simulink model "Motor_Control_STR"  (R2022a)
settings: Solver=FixedStepDiscrete  StartTime=0.0  StopTime=200  FixedStep=0.005  RelTol=1e-3
libraries: slpidlib x1
settings Model: Creator=PC  LastModifiedBy=dat
settings SolverCC: AlgebraicLoopSolver=TrustRegion
settings DataIOCC: ReturnWorkspaceOutputs=off
settings OptimizationCC: DefaultParameterBehavior=Inlined  PassReuseOutputArgsAs=Individual arguments  EfficientTunableParamExpr=on
settings DebuggingCC: ParameterTunabilityLossMsg=error  UnconnectedInputMsg=warning  UnconnectedOutputMsg=warning  UnconnectedLineMsg=warning  ArithmeticOperatorsInVariantConditions=warning
settings SFSimCC: SimUseLocalCustomCode=off  MATLABDynamicMemAlloc=off  CustomCodeUndefinedFunction=UseInterfaceOnly
settings RTWCC: SystemTargetFile=ert.tlc  GenCodeOnly=on  TemplateMakefile=ert_default_tmf  GenerateReport=on  RTWUseLocalCustomCode=off  IncludeHyperlinkInReport=on  LaunchReport=on  GenerateTraceInfo=on  GenerateTraceReport=on  GenerateTraceReportSl=on  GenerateTraceReportSf=on  GenerateTraceReportEml=on
settings CodeAppCC: ForceParamTrailComments=on  IgnoreCustomStorageClasses=off  OperatorAnnotations=on  SimulinkDataObjDesc=on  SFDataObjDesc=on  InsertBlockDesc=on
settings ERTTargetCC: TargetLangStandard=C99 (ISO)  GenerateSampleERTMain=on  InlinedParameterPlacement=NonHierarchical  ERTCustomFileTemplate=example_file_process.tlc

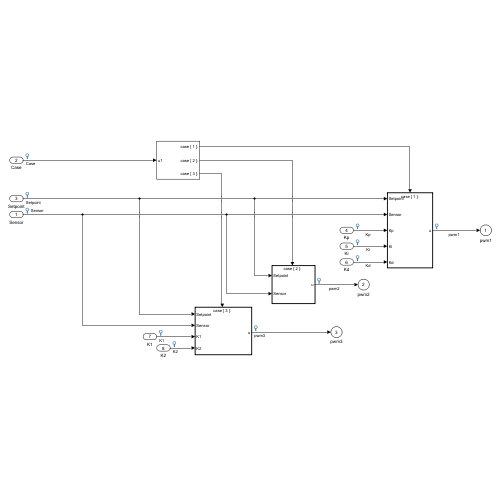
[thumbnail: Simulink's stored preview of the top-level diagram]
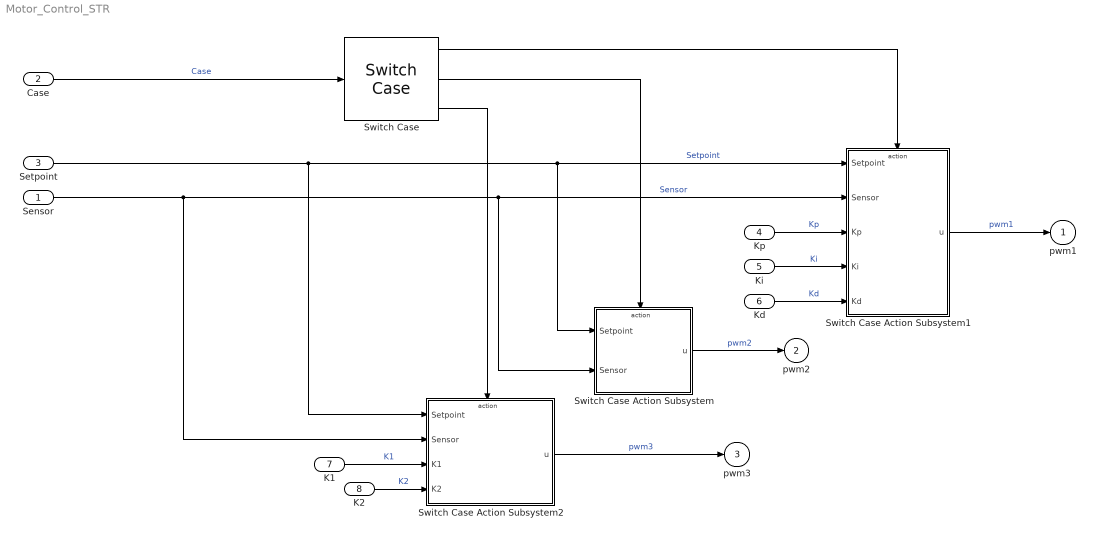
== system Motor_Control_STR ==
  Sensor : Inport
  Case : Inport  Port=2
  Setpoint : Inport  Port=3
  Kp : Inport  Port=4
  Ki : Inport  Port=5
  Kd : Inport  Port=6
  K1 : Inport  Port=7
  K2 : Inport  Port=8
  Switch Case : SwitchCase  CaseConditions={1,2,3}  ShowDefaultCase=off
  Switch Case Action Subsystem : Subsystem  TreatAsAtomicUnit=on
  Switch Case Action Subsystem1 : Subsystem  TreatAsAtomicUnit=on
  Switch Case Action Subsystem2 : Subsystem  TreatAsAtomicUnit=on
  pwm1 : Outport  VectorParamsAs1DForOutWhenUnconnected=off
  pwm2 : Outport  Port=2  VectorParamsAs1DForOutWhenUnconnected=off
  pwm3 : Outport  Port=3  VectorParamsAs1DForOutWhenUnconnected=off
  wires:
  Case/1 -> Switch Case/1  "Case"
  Sensor/1 -> Switch Case Action Subsystem2/2(Sensor), Switch Case Action Subsystem/2(Sensor), Switch Case Action Subsystem1/2(Sensor)  "Sensor"
  Switch Case Action Subsystem1/1(u) -> pwm1/1  "pwm1"
  Switch Case/2 -> Switch Case Action Subsystem/Action
  Switch Case/1 -> Switch Case Action Subsystem1/Action
  Kp/1 -> Switch Case Action Subsystem1/3(Kp)  "Kp"
  Ki/1 -> Switch Case Action Subsystem1/4(Ki)  "Ki"
  Kd/1 -> Switch Case Action Subsystem1/5(Kd)  "Kd"
  Setpoint/1 -> Switch Case Action Subsystem2/1(Setpoint), Switch Case Action Subsystem/1(Setpoint), Switch Case Action Subsystem1/1(Setpoint)  "Setpoint"
  Switch Case Action Subsystem/1(u) -> pwm2/1  "pwm2"
  Switch Case Action Subsystem2/1(u) -> pwm3/1  "pwm3"
  Switch Case/3 -> Switch Case Action Subsystem2/Action
  K2/1 -> Switch Case Action Subsystem2/4(K2)  "K2"
  K1/1 -> Switch Case Action Subsystem2/3(K1)  "K1"

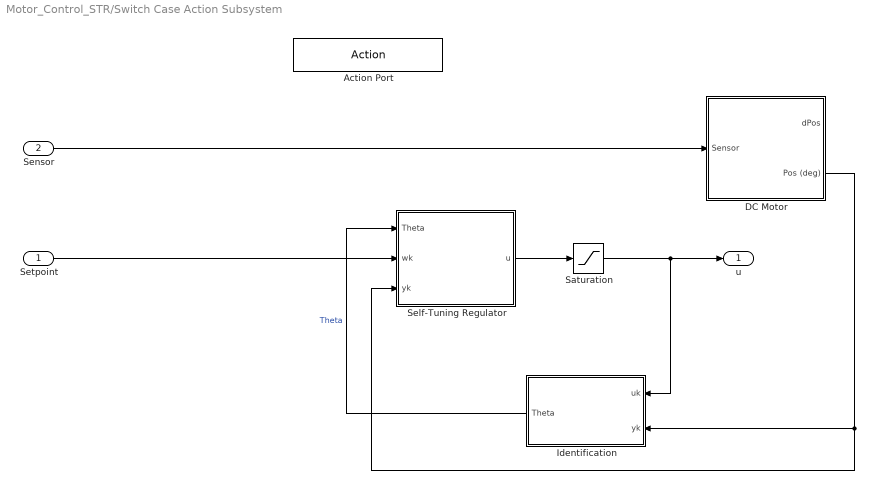
== system Motor_Control_STR/Switch Case Action Subsystem ==
  Setpoint : Inport
  Sensor : Inport  Port=2
  Action Port : ActionPort  ActionPortLabel=case [ 2 ]:
  DC Motor : Subsystem
  Identification : Subsystem
  Saturation : Saturate  UpperLimit=10  LowerLimit=-10
  Self-Tuning Regulator : Subsystem
  u : Outport  VectorParamsAs1DForOutWhenUnconnected=off
  wires:
  Setpoint/1 -> Self-Tuning Regulator/2(wk)
  DC Motor/2(Pos (deg)) -> Self-Tuning Regulator/3(yk), Identification/2(yk)
  Sensor/1 -> DC Motor/1(Sensor)
  Identification/1(Theta) -> Self-Tuning Regulator/1(Theta)  "Theta"
  Self-Tuning Regulator/1(u) -> Saturation/1
  Saturation/1 -> u/1, Identification/1(uk)

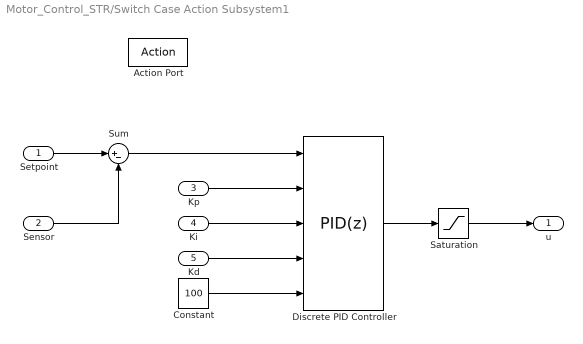
== system Motor_Control_STR/Switch Case Action Subsystem1 ==
  Setpoint : Inport
  Sensor : Inport  Port=2
  Kp : Inport  Port=3
  Ki : Inport  Port=4
  Kd : Inport  Port=5
  Action Port : ActionPort  ActionPortLabel=case [ 1 ]:
  Constant : Constant  Value=100
  Discrete PID Controller : slpidlib/PID Controller  Controller=PID  Form=Parallel  TimeDomain=Discrete-time  UseExternalTs=off  SampleTime=-1  IntegratorMethod=Forward Euler  FilterMethod=Forward Euler  ControllerParametersSource=external  P=1  I=1  UseKiTs=off  D=0  N=100  UseFilter=on  TunerSelectOption=Transfer Function Based (PID Tuner App)  InitialConditionSource=internal  InitialConditionForIntegrator=0  InitialConditionForFilter=0  DifferentiatorICPrevScaledInput=0  ExternalReset=none  TrackingMode=off  Kt=1  LimitOutput=off  SatLimitsSource=internal  UpperSaturationLimit=inf  LowerSaturationLimit=-inf  LinearizeAsGain=off  AntiWindupMode=none  Kb=1  POutMin=[]  POutMax=[]  IOutMin=[]  IOutMax=[]  DOutMin=[]  DOutMax=[]  NOutMin=[]  NOutMax=[]  SumOutMin=[]  SumOutMax=[]  SaturationOutMin=[]  SaturationOutMax=[]  PParamMin=[]  PParamMax=[]  IParamMin=[]  IParamMax=[]  DParamMin=[]  DParamMax=[]  NParamMin=[]  NParamMax=[]  KbParamMin=[]  KbParamMax=[]  KtParamMin=[]  KtParamMax=[]  KbOutMin=[]  KbOutMax=[]  KtOutMin=[]  KtOutMax=[]  IntegratorOutMin=[]  IntegratorOutMax=[]  FilterOutMin=[]  FilterOutMax=[]  SumI1OutMin=[]  SumI1OutMax=[]  SumI2OutMin=[]  SumI2OutMax=[]  SumI3OutMin=[]  SumI3OutMax=[]  SumI4OutMin=[]  SumI4OutMax=[]  SumDOutMin=[]  SumDOutMax=[]  DifferentiatorOutMin=[]  DifferentiatorOutMax=[]  FilterDiffOutCoefMin=[]  FilterDiffOutCoefMax=[]  ReciprocalOutMin=[]  ReciprocalOutMax=[]  SumDenOutMin=[]  SumDenOutMax=[]  SumNumOutMin=[]  SumNumOutMax=[]  DivideOutMin=[]  DivideOutMax=[]  UdiffTsProdOutMin=[]  UdiffTsProdOutMax=[]  NTsProdOutMin=[]  NTsProdOutMax=[]  UintegralTsProdOutMin=[]  UintegralTsProdOutMax=[]  UngainTsProdOutMin=[]  UngainTsProdOutMax=[]  IntegratorContinuousStateAttributes=''  IntegratorStateMustResolveToSignalObject=off  IntegratorRTWStateStorageClass=Auto  FilterContinuousStateAttributes=''  FilterStateMustResolveToSignalObject=off  FilterRTWStateStorageClass=Auto  ParallelPVariant=ExternalParameters  IdealPVariant=Disabled  IVariant=ExternalParameters  DVariant=ExternalParameters  IntegratorVariant=Discrete  SatVariant=Disabled  AWVariant=Passthrough  PCopyVariant=Disabled  TRVariant=Disabled  FdbkBlocksVariant=Forward  IdealPFdbkVariant=Disabled  SatFdbkVariant=Disabled  DerivativeFilterVariant=ForwardEulerFilter  NVariant=ExternalParameters  NCopyVariant=Disabled  FilterICVariant=InternalICsFilter  IntegratorICVariant=InternalICs  ExternalResetVariant=Disabled  TRSumVariant=Passthrough  SumFdbkVariant=Disabled  SumVariant=Sum_PID  TsampFilterVariant=InternalTs  TsampNgainVariant=Passthrough  TsampIntegralVariant=Disabled_SignalSpec  ExternalSaturationOutDataTypeStr=Inherit: Same as second input
  Saturation : Saturate  UpperLimit=10  LowerLimit=-10
  Sum : Sum  Inputs=|+-
  u : Outport  VectorParamsAs1DForOutWhenUnconnected=off
  wires:
  Setpoint/1 -> Sum/1
  Sensor/1 -> Sum/2
  Sum/1 -> Discrete PID Controller/1
  Kp/1 -> Discrete PID Controller/2
  Ki/1 -> Discrete PID Controller/3
  Kd/1 -> Discrete PID Controller/4
  Constant/1 -> Discrete PID Controller/5
  Discrete PID Controller/1 -> Saturation/1
  Saturation/1 -> u/1

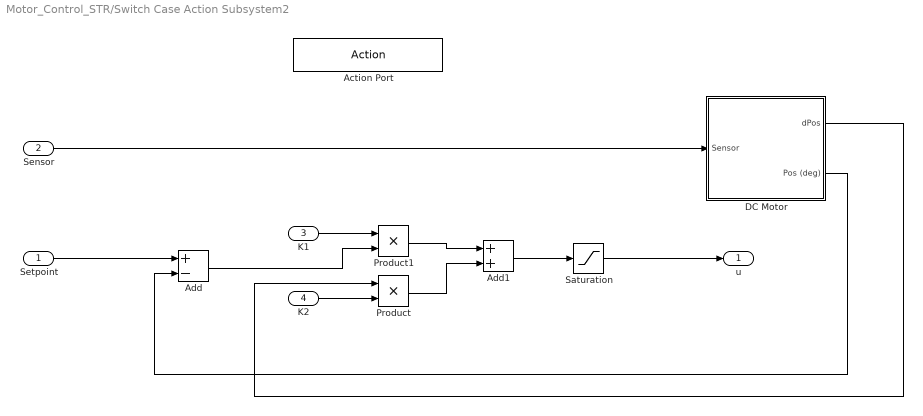
== system Motor_Control_STR/Switch Case Action Subsystem2 ==
  Setpoint : Inport
  Sensor : Inport  Port=2
  K1 : Inport  Port=3
  K2 : Inport  Port=4
  Action Port : ActionPort  ActionPortLabel=case [ 3 ]:
  Add : Sum  Inputs=+-
  Add1 : Sum
  DC Motor : Subsystem
  Product : Product
  Product1 : Product
  Saturation : Saturate  UpperLimit=10  LowerLimit=-10
  u : Outport  VectorParamsAs1DForOutWhenUnconnected=off
  wires:
  Sensor/1 -> DC Motor/1(Sensor)
  Add1/1 -> Saturation/1
  Saturation/1 -> u/1
  Setpoint/1 -> Add/1
  DC Motor/2(Pos (deg)) -> Add/2
  K1/1 -> Product1/1
  Add/1 -> Product1/2
  K2/1 -> Product/2
  DC Motor/1(dPos) -> Product/1
  Product1/1 -> Add1/1
  Product/1 -> Add1/2

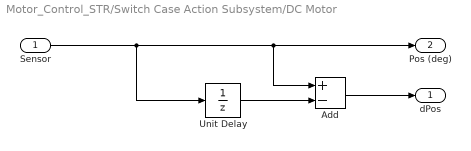
== system Motor_Control_STR/Switch Case Action Subsystem/DC Motor ==
  Sensor : Inport
  Add : Sum  Inputs=+-
  Unit Delay : UnitDelay  SampleTime=-1  HasFrameUpgradeWarning=on
  dPos : Outport  VectorParamsAs1DForOutWhenUnconnected=off
  Pos (deg) : Outport  Port=2  VectorParamsAs1DForOutWhenUnconnected=off
  wires:
  Unit Delay/1 -> Add/2
  Sensor/1 -> Unit Delay/1, Pos (deg)/1, Add/1
  Add/1 -> dPos/1

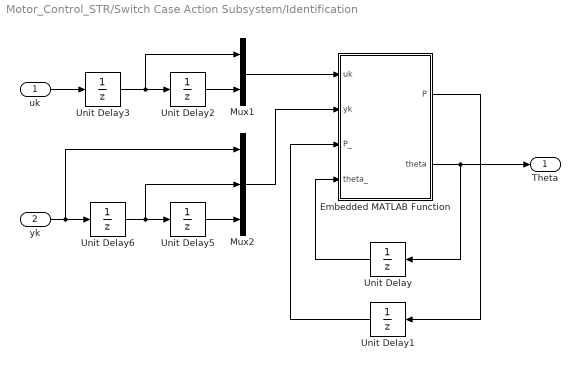
== system Motor_Control_STR/Switch Case Action Subsystem/Identification ==
  uk : Inport  PortDimensions=1
  yk : Inport  Port=2  PortDimensions=1
  Embedded MATLAB Function : MATLAB Function  TreatAsAtomicUnit=on
  Mux1 : Mux  Inputs=2
  Mux2 : Mux  Inputs=3
  Unit Delay : UnitDelay  InitialCondition=[-1; 0.1; 0.1; 1]  SampleTime=-1  HasFrameUpgradeWarning=on
  Unit Delay1 : UnitDelay  InitialCondition=1e5*eye(4)  SampleTime=-1  HasFrameUpgradeWarning=on
  Unit Delay{2..3,5..6} (4 alike) : UnitDelay  SampleTime=-1  HasFrameUpgradeWarning=on
  Theta : Outport  PortDimensions=4  VectorParamsAs1DForOutWhenUnconnected=off
  wires:
  Unit Delay/1 -> Embedded MATLAB Function/4(theta_)
  Embedded MATLAB Function/2(theta) -> Unit Delay/1, Theta/1
  Unit Delay1/1 -> Embedded MATLAB Function/3(P_)
  Embedded MATLAB Function/1(P) -> Unit Delay1/1
  Mux1/1 -> Embedded MATLAB Function/1(uk)
  Unit Delay6/1 -> Mux2/2, Unit Delay5/1
  Unit Delay5/1 -> Mux2/3
  Mux2/1 -> Embedded MATLAB Function/2(yk)
  Unit Delay2/1 -> Mux1/2
  Unit Delay3/1 -> Unit Delay2/1, Mux1/1
  uk/1 -> Unit Delay3/1
  yk/1 -> Unit Delay6/1, Mux2/1

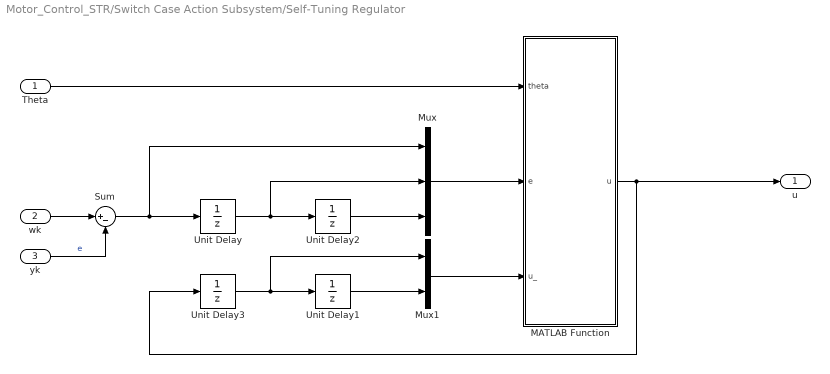
== system Motor_Control_STR/Switch Case Action Subsystem/Self-Tuning Regulator ==
  Theta : Inport
  wk : Inport  Port=2
  yk : Inport  Port=3
  MATLAB Function : MATLAB Function  TreatAsAtomicUnit=on
  Mux : Mux  Inputs=3
  Mux1 : Mux  Inputs=2
  Sum : Sum  Inputs=|+-
  Unit Delay{,1..3} (4 alike) : UnitDelay  SampleTime=-1  HasFrameUpgradeWarning=on
  u : Outport  VectorParamsAs1DForOutWhenUnconnected=off
  wires:
  Unit Delay/1 -> Mux/2, Unit Delay2/1
  Unit Delay2/1 -> Mux/3
  Theta/1 -> MATLAB Function/1(theta)
  Mux1/1 -> MATLAB Function/3(u_)
  Unit Delay1/1 -> Mux1/2
  Unit Delay3/1 -> Mux1/1, Unit Delay1/1
  MATLAB Function/1(u) -> Unit Delay3/1, u/1
  Mux/1 -> MATLAB Function/2(e)
  Sum/1 -> Mux/1, Unit Delay/1
  wk/1 -> Sum/1
  yk/1 -> Sum/2  "e"

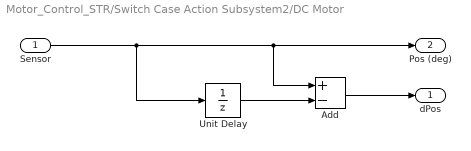
== system Motor_Control_STR/Switch Case Action Subsystem2/DC Motor ==
  Sensor : Inport
  Add : Sum  Inputs=+-
  Unit Delay : UnitDelay  SampleTime=-1  HasFrameUpgradeWarning=on
  dPos : Outport  VectorParamsAs1DForOutWhenUnconnected=off
  Pos (deg) : Outport  Port=2  VectorParamsAs1DForOutWhenUnconnected=off
  wires:
  Unit Delay/1 -> Add/2
  Sensor/1 -> Unit Delay/1, Pos (deg)/1, Add/1
  Add/1 -> dPos/1

== matlab function Motor_Control_STR/Switch Case Action Subsystem/Self-Tuning Regulator/MATLAB Function ==
  data: theta input; u output; e input; u_ input
function u = STR_pp1(theta,e,u_)
% Cai dat thoi gian lay mau va cuc mong muon
T0 = 0.005;
xi = 0.99;
wn = 4;
 
% Gan lai cho de su dung
a1   =  theta(1);
a2   =  theta(2);
b1   =  theta(3);
b2   =  theta(4);
 
% Sinh vien viet bo sung doan code phan dieu khien
 
if( xi<1)
    d1 = -2*exp(-xi*wn*T0)*cos(wn*T0*sqrt(1-xi^2));
else
    d1 = -2*exp(-xi*wn*T0)*cosh(wn*T0*sqrt(xi^2-1));
end
 
d2 = exp(-2*xi*wn*T0);
 
r1 = (b1+b2)*(a1*b1*b2-a2*b1^2-b2^2);
s1 = a2*((b1+b2)*(a1*b2-a2*b1)+b2*(b1*d2-b2*d1-b2));
q2 = s1/r1;
gamma = q2*b2/a2;
q1 = (a2/b2)-q2*(b1/b2-a1/a2+1);
q0 = (d1+1-a1-gamma)/b1;
 
%control law
u = q0*e(1) + q1*e(2) + q2*e(3) + (1-gamma)*u_(1) + gamma*u_(2);

== matlab function Motor_Control_STR/Switch Case Action Subsystem/Identification/Embedded MATLAB Function ==
  settings: fimath=|
      | fimath(...
      | 'RoundMode', 'floor',...
      | 'OverflowMode', 'wrap',...
      | 'ProductMode', 'KeepLSB', 'ProductWordLength', 32,...
      | 'SumMode', 'KeepLSB', 'SumWordLength', 32,...
      | 'CastBeforeSum', false)
  data: P output; uk input; yk input; P_ input; theta_ input; theta output
function [P,theta] = Uocluong(uk,yk,P_,theta_)
lamda = 0.99;
PHI = [-yk(2); -yk(3); uk(1); uk(2)];
e = yk(1) - PHI'*theta_;
L = P_*PHI / (lamda + PHI'*P_*PHI);
P = 1/lamda*(P_ - P_*PHI*PHI'*P_ /(lamda + PHI'*P_*PHI));
theta = theta_ + L*e;
